simulink model "DOUBLE_Pendulum_Linear"  (R2019b)
settings: Solver=ode45  StartTime=0.0  StopTime=13.0  RelTol=1e-6  EnableMultiTasking=on
InitFcn:
  | L1= 5; L2 = L1;      % m
  | g = 9.81;            % m/s^2
  | m1=10;               % kg
  | m2=10;               % kg
  | M=m1+m2;
settings Model: Creator=David  LastModifiedBy=sulaymon.eshkabilov
settings OptimizationCC: ExpressionDepthLimit=2147483647  LifeSpan=inf
settings DebuggingCC: UnderspecifiedInitializationDetection=Classic  MergeDetectMultiDrivingBlocksExec=none  SolverPrmCheckMsg=warning  StateNameClashWarn=warning  SFUnexpectedBacktrackingDiag=warning  SFNoUnconditionalDefaultTransitionDiag=warning  SFExecutionAtInitializationDiag=none  ArithmeticOperatorsInVariantConditions=warning
settings HardwareCC: ProdBitPerPointer=32  ProdBitPerSizeT=32  ProdBitPerPtrDiffT=32  ProdLargestAtomicFloat=None  ProdIntDivRoundTo=Undefined  ProdEndianess=Unspecified  ProdWordSize=32  ProdHWDeviceType=32-bit Generic
settings ModelReferenceCC: PropagateSignalLabelsOutOfModel=off
settings SFSimCC: SimUseLocalCustomCode=off  CustomCodeUndefinedFunction=UseInterfaceOnly
settings RTWCC: RTWUseLocalCustomCode=off
settings CodeAppCC: StateflowObjectComments=on
settings GRTTargetCC: TargetLangStandard=C89/C90 (ANSI)  GeneratePreprocessorConditionals=Disable all
settings ConfigComp: CovMetricSettings=dw  CovHtmlReporting=on  CovSaveCumulativeToWorkspaceVar=on  CovSaveSingleToWorkspaceVar=on  CovExternalEMLEnable=off

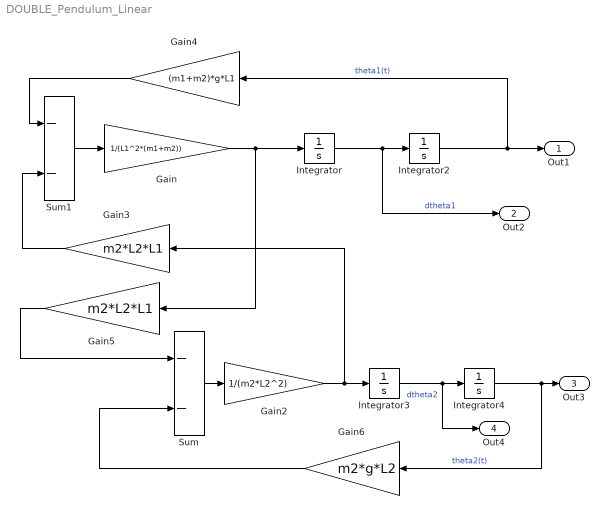
== system DOUBLE_Pendulum_Linear ==
  Gain : Gain  Gain=1/(L1^2*(m1+m2))
  Gain2 : Gain  Gain=1/(m2*L2^2)
  Gain3 : Gain  Gain=m2*L2*L1
  Gain4 : Gain  Gain=(m1+m2)*g*L1
  Gain5 : Gain  Gain=m2*L2*L1
  Gain6 : Gain  Gain=m2*g*L2
  Integrator : Integrator  InitialCondition=-1
  Integrator2 : Integrator  InitialCondition=-.5
  Integrator3 : Integrator  InitialCondition=2
  Integrator4 : Integrator  InitialCondition=1
  Sum : Sum  RequirementInfo={} %GIDa_6605b2c0_cc9d_4c7f_bc18_75536daf65c1  Inputs=--
  Sum1 : Sum  Inputs=--
  Out1 : Outport
  Out2 : Outport  Port=2
  Out3 : Outport  Port=3
  Out4 : Outport  Port=4
  wires:
  Integrator2/1 -> Out1/1, Gain4/1  "theta1(t)"
  Gain2/1 -> Integrator3/1, Gain3/1
  Integrator3/1 -> Integrator4/1, Out4/1  "dtheta2"
  Integrator4/1 -> Out3/1, Gain6/1  "theta2(t)"
  Sum1/1 -> Gain/1
  Sum/1 -> Gain2/1
  Gain3/1 -> Sum1/2
  Gain4/1 -> Sum1/1
  Integrator/1 -> Out2/1, Integrator2/1  "dtheta1"
  Gain/1 -> Gain5/1, Integrator/1
  Gain5/1 -> Sum/1
  Gain6/1 -> Sum/2
